simulink model "Part2_DiscreteEvent"  (R2024b)
settings: Solver=ode1  StartTime=0.0  StopTime=15  FixedStep=0.001  RelTol=1e-3
settings Model: Creator=SherOu  LastModifiedBy=SherOu

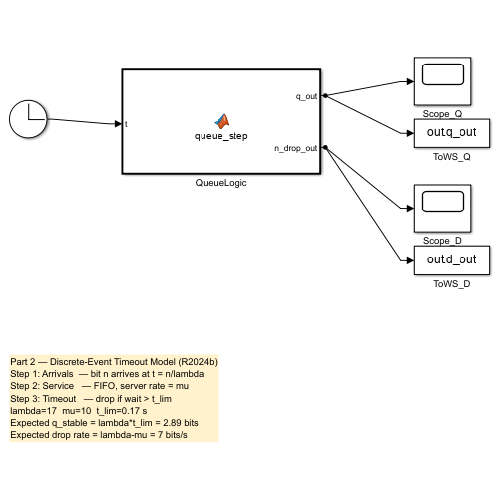
[thumbnail: Simulink's stored preview of the top-level diagram]
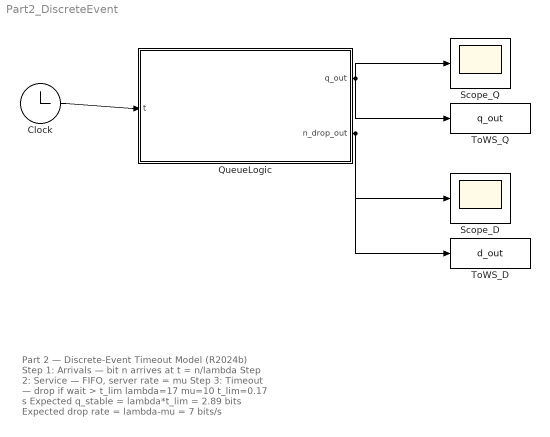
== system Part2_DiscreteEvent ==
  note: Part 2 — Discrete-Event Timeout Model (R2024b)
      | Step 1: Arrivals  — bit n arrives at t = n/lambda
      | Step 2: Service   — FIFO, server rate = mu
      | Step 3: Timeout   — drop if wait > t_lim
      | lambda=17  mu=10  t_lim=0.17 s
      | Expected q_stable = lambda*t_lim = 2.89 bits
      | Expected drop rate = lambda-mu = 7 bits/s
  Clock : Clock
  QueueLogic : MATLAB Function  TreatAsAtomicUnit=on
  Scope_D : Scope
  Scope_Q : Scope
  ToWS_D : ToWorkspace  VariableName=d_out  SampleTime=-1
  ToWS_Q : ToWorkspace  VariableName=q_out  SampleTime=-1
  wires:
  Clock/1 -> QueueLogic/1(t)
  QueueLogic/1(q_out) -> Scope_Q/1, ToWS_Q/1
  QueueLogic/2(n_drop_out) -> Scope_D/1, ToWS_D/1

== matlab function Part2_DiscreteEvent/QueueLogic ==
  data: t input; q_out output; n_drop_out output
function [q_out, n_drop_out] = queue_step(t)
% Discrete-event FIFO queue with timeout
% Ported from Julia: arrivals -> service -> timeout
% lambda=17.0  mu=10.0  t_lim=0.1700

    persistent n_arr n_drop buffer buf_size server_busy_until

    LAMBDA  = 17.0;     % bits/s arrival rate
    MU      = 10.0;     % bits/s service rate
    T_LIM   = 0.1700;  % seconds timeout
    MAX_BUF = 2000;    % pre-allocated buffer size

    if isempty(n_arr)
        n_arr             = 0.0;
        n_drop            = 0.0;
        buffer            = zeros(1, MAX_BUF);
        buf_size          = 0.0;
        server_busy_until = 0.0;
    end

    % STEP 1 - Arrivals
    % Bit n_arr arrives at t = n_arr/LAMBDA (uniform stream)
    % Add all bits that have arrived by current time t
    while n_arr / LAMBDA <= t
        buf_size          = buf_size + 1;
        buffer(buf_size)  = n_arr / LAMBDA;  % store arrival time
        n_arr             = n_arr + 1;
    end

    % STEP 2 - Server processing
    % While server is free, serve the oldest bit (FIFO)
    while buf_size > 0 && server_busy_until <= t
        start_time        = max(t, buffer(1));
        server_busy_until = start_time + 1.0 / MU;
        if buf_size > 1
            buffer(1:buf_size-1) = buffer(2:buf_size);
        end
        buf_size = buf_size - 1;
    end

    % STEP 3 - Timeout check
    % Drop oldest bit if it has waited longer than T_LIM
    while buf_size > 0 && (t - buffer(1)) > T_LIM
        if buf_size > 1
            buffer(1:buf_size-1) = buffer(2:buf_size);
        end
        buf_size = buf_size - 1;
        n_drop   = n_drop + 1;
    end

    q_out      = buf_size;   % current buffer length
    n_drop_out = n_drop;     % cumulative dropped bits
end
